simulink model "practica6"  (R2019b)
settings: Solver=VariableStepAuto  StartTime=0.0  StopTime=10.0  RelTol=1e-3
undefined symbols (not defined in the file): boton, sensor, sonar
libraries: legoev3lib x9
settings Model: Creator=alumnopr09  LastModifiedBy=alumnopr09

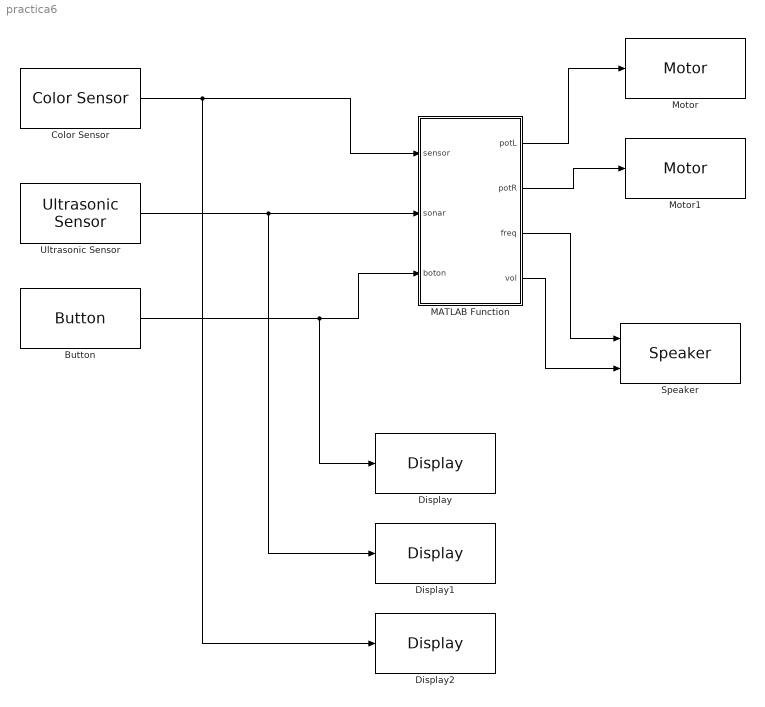
== system practica6 ==
  Button : legoev3lib/Button  buttonType=Up  sampleTime=0.1
      settings: SourceProductName=Simulink Support Package for LEGO MINDSTORMS EV3 Hardware  SourceProductBaseCode=LEGOEV3
  Color Sensor : legoev3lib/Color Sensor  portNumber=1  mode=Reflected light intensity  sampleTime=0.1
      settings: SourceProductName=Simulink Support Package for LEGO MINDSTORMS EV3 Hardware  SourceProductBaseCode=LEGOEV3
  Display : legoev3lib/Display  slcdStr=boton:  slcdLine=1  slcdFormat=Decimal
      settings: SourceProductName=Simulink Support Package for LEGO MINDSTORMS EV3 Hardware  SourceProductBaseCode=LEGOEV3
  Display1 : legoev3lib/Display  slcdStr=sonar:  slcdLine=2  slcdFormat=Decimal
      settings: SourceProductName=Simulink Support Package for LEGO MINDSTORMS EV3 Hardware  SourceProductBaseCode=LEGOEV3
  Display2 : legoev3lib/Display  slcdStr=sensor:  slcdLine=3  slcdFormat=Decimal
      settings: SourceProductName=Simulink Support Package for LEGO MINDSTORMS EV3 Hardware  SourceProductBaseCode=LEGOEV3
  MATLAB Function : MATLAB Function  TreatAsAtomicUnit=on
  Motor : legoev3lib/Motor  sportNumber=A  sstopAction=Brake
  Motor1 : legoev3lib/Motor  sportNumber=A  sstopAction=Brake
  Speaker : legoev3lib/Speaker  sinputMode=Frequency and volume  sspeakerFreq=100  sspeakerVolume=50  sspeakerDuration=100
      settings: SourceProductName=Simulink Support Package for LEGO MINDSTORMS EV3 Hardware  SourceProductBaseCode=LEGOEV3
  Ultrasonic Sensor : legoev3lib/Ultrasonic Sensor  PortNumber=1  sampleTime=0.1
      settings: SourceProductName=Simulink Support Package for LEGO MINDSTORMS EV3 Hardware  SourceProductBaseCode=LEGOEV3
  wires:
  Ultrasonic Sensor/1 -> Display1/1, MATLAB Function/2(sonar)
  Color Sensor/1 -> Display2/1, MATLAB Function/1(sensor)
  Button/1 -> Display/1, MATLAB Function/3(boton)
  MATLAB Function/1(potL) -> Motor/1
  MATLAB Function/2(potR) -> Motor1/1
  MATLAB Function/3(freq) -> Speaker/1
  MATLAB Function/4(vol) -> Speaker/2

== matlab function practica6/MATLAB Function ==
  data: sensor input; potL output; sonar input; boton input; potR output; freq output; vol output
function [potL, potR, freq, vol] = main(sensor, sonar, boton)
p = 50; % potencia motores


% estado = true --> buscar
% estado = false --> parado
persistent estado 
if (isempty(estado))
    estado = true;
end


if (estado) % no he encontrado nada
    % Compruebo si veo un papel
    detected = Foraging(sensor);
    if (detected) % Detecto algo
        estado = false;
    else % Sigo sin ver nada
        % Compruebo si tengo obstaculo
        ignore, pl, pr = ObstacleAvoidance(sonar,p);
        if (ignore) % Deambulamos
            % Movimientos aleatorios
            pl, pr = Wandering(pl,pr);      
        end
        potL = pl;
        potR = pr;
        estado = true; % Redundante

    end    
else % he encontrado algo
    freq = 1000; % in Hz
    vol = 1; % from 0 to 100
    % boton = 0 --> Not pressed
    % boton = 1 --> Pressed
    if (boton)
        estado = true;
    end
end

%-------------------------------
% Estado del robot y del altavoz
%-------------------------------
function detected = Foraging(sensor)
umbral_luz = 50;

if (sensor > umbral_luz) % ha encontrado un objeto
    detected = true;
    
else % no he encontrado nada
    detected = false;
end

%-----------------------------------
% Deteccion obstaculos y pot motores
%-----------------------------------
function ignore, pl, pr = ObstacleAvoidance(sonar)
umbral_dist = 35; %cm

if (sonar < umbral_dist) 
   pl = -p; 
   pr = -p;
   
end

%---------------------------------
% Movimientos aleatorios del robot
%---------------------------------
function Wandering(pl, pr)
    
y = u
